simulink model "Task4_sim"  (R2024b)
settings: Solver=ode4  StartTime=0.0  StopTime=100  FixedStep=0.1  RelTol=1e-3
values from neighbouring files (symbols this model uses):
  I = diag([Ix, Iy, Iz])    [Task1.m]    (also in Task2.m; Task3.m; Task4.m)
  Ir = 0.0050    (= 0.005)    [Task4.m]
  Ix = 0.0700    (= 0.07)    [Task1.m]    (also in Task2.m = 0.0504; Task3.m = 0.025; Task4.m)
  Iy = 0.055    [Task1.m]    (also in Task2.m = 0.0504; Task3.m; Task4.m = 0.0109)
  Iz = 0.025    [Task1.m]    (also in Task2.m = 0.0109; Task3.m = 0.07; Task4.m = 0.0504)
  w_0 = [0.45, 0.52, 0.52]'    [Task1.m]    (also in Task2.m = [wx_0, wy_0, wz_0]'; Task3.m = [0.1, 0.1, 2]'; Task4.m = [1e-6, 1e-6, 0.02]')
  wr_0 = 2*pi    (= 6.28318530718)    [Task4.m]
libraries: matrix_library x1
settings Model: Creator=alejandromunozvazquez  LastModifiedBy=alejandromunozvazquez

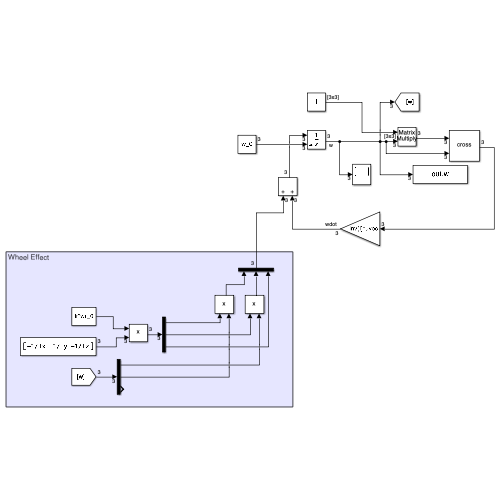
[thumbnail: Simulink's stored preview of the top-level diagram]
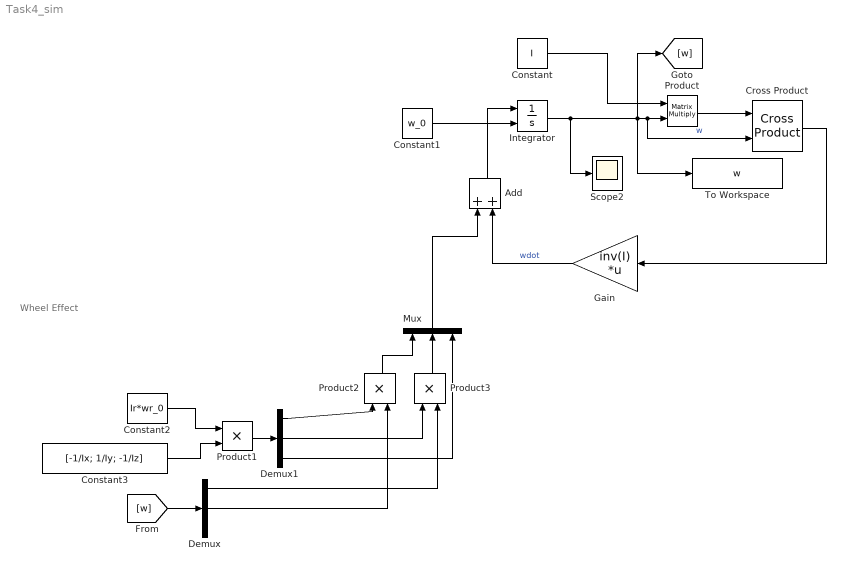
== system Task4_sim ==
  note: Wheel Effect
  Add : Sum
  Constant : Constant  Value=I
  Constant1 : Constant  Value=w_0
  Constant2 : Constant  Value=Ir*wr_0
  Constant3 : Constant  Value=[-1/Ix; 1/Iy; -1/Iz]
  Cross Product : matrix_library/Cross Product
  Demux : Demux  Outputs=3
  Demux1 : Demux  Outputs=3
  Gain : Gain  Gain=inv(I)  Multiplication=Matrix(K*u) (u vector)
  Integrator : Integrator  InitialConditionSource=external
  Mux : Mux  Inputs=3
  Product : Product  Multiplication=Matrix(*)
  Product1 : Product
  Product2 : Product
  Product3 : Product
  Scope2 : Scope
  To Workspace : ToWorkspace  VariableName=w  SampleTime=-1
  wires:
  Integrator/1 -> [w], Product/2, Cross Product/2, To Workspace/1, Scope2/1  "w"
  Constant/1 -> Product/1
  Product/1 -> Cross Product/1
  Cross Product/1 -> Gain/1
  Constant1/1 -> Integrator/2
  Add/1 -> Integrator/1
  Gain/1 -> Add/2  "wdot"
  Constant2/1 -> Product1/1
  Constant3/1 -> Product1/2
  [w] -> Demux/1
  Product1/1 -> Demux1/1
  Demux/1 -> Product3/2
  Demux/2 -> Product2/2
  Demux1/1 -> Product2/1
  Demux1/2 -> Product3/1
  Product3/1 -> Mux/2
  Product2/1 -> Mux/1
  Mux/1 -> Add/1
  Demux1/3 -> Mux/3
